simulink model "PCM"  (R2024a)
settings: Solver=VariableStepAuto  StartTime=0.0  StopTime=10.0  RelTol=1e-3
values from neighbouring files (symbols this model uses):
  C = 200*10^(-6)    (= 0.0002)    [Parameters.m]
  ESR = .8    (= 0.8)    [Parameters.m]
  Fs = 10*10^(6)    (= 10000000)    [Parameters.m]
  L = 1*10^(-6)    (= 1e-06)    [Parameters.m]
  Rf = .1    (= 0.1)    [Parameters.m]
  RL = 15*10^(-3)    (= 0.015)    [Parameters.m]
  Rload = 1000    [Parameters.m]
libraries: spsSeriesRLCBranchLib x4, spsMosfetLib x2, spsControlledCurrentSourceLib x1, spsDCVoltageSourceLib x1, simulink_extras x1, spsStairGeneratorLib x1, spsVoltageMeasurementLib x1
settings Model: Creator=User  LastModifiedBy=User

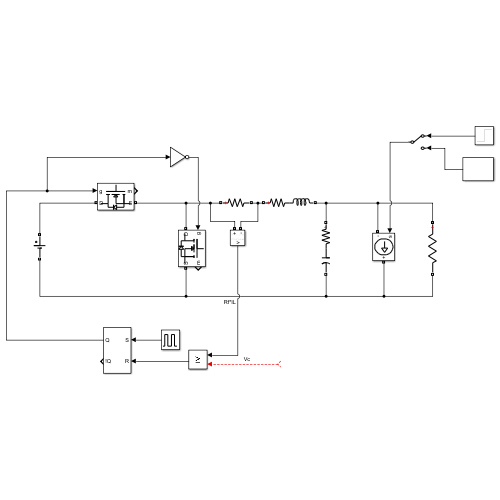
[thumbnail: Simulink's stored preview of the top-level diagram]
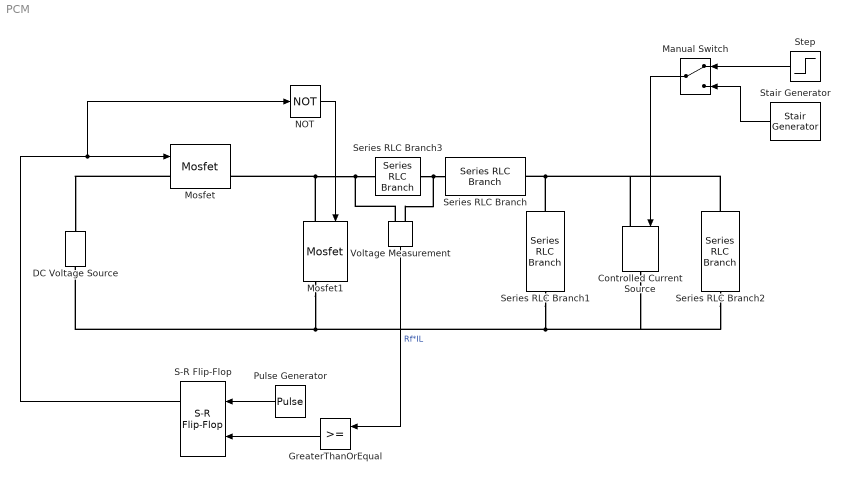
== system PCM ==
  Controlled Current Source : spsControlledCurrentSourceLib/Controlled Current Source  Initialize=on  Source_Type=AC  Amplitude=0  Phase=0  Frequency=0  Measurements=None
  DC Voltage Source : spsDCVoltageSourceLib/DC Voltage Source  Amplitude=5  Measurements=None
  GreaterThanOrEqual : RelationalOperator  OutDataTypeStr=boolean  RndMeth=Simplest  InputSameDT=off
  Manual Switch : ManualSwitch
  Mosfet : spsMosfetLib/Mosfet  Ron=0.1  Lon=0  Rd=0.01  Vfd=0  IC=0  Rs=1e5  Cs=inf  Measurements=on
  Mosfet1 : spsMosfetLib/Mosfet  Ron=0.1  Lon=0  Rd=0.01  Vfd=0  IC=0  Rs=1e5  Cs=inf  Measurements=on
  NOT : Logic  Operator=NOT  IconShape=distinctive  AllPortsSameDT=off  OutDataTypeStr=boolean
  Pulse Generator : DiscretePulseGenerator  PulseType=Time based  Period=1/Fs  PulseWidth=10
  S-R Flip-Flop : simulink_extras/Flip Flops/S-R Flip-Flop  initial_condition=0
  Series RLC Branch : spsSeriesRLCBranchLib/Series RLC Branch  LConnTagsString=__new0  RConnTagsString=__new0  BranchType=RL  Resistance=RL  Inductance=L  SetiL0=off  InitialCurrent=0  Capacitance=1e-6  Setx0=off  InitialVoltage=0  Measurements=None
  Series RLC Branch1 : spsSeriesRLCBranchLib/Series RLC Branch  LConnTagsString=__new0  RConnTagsString=__new0  BranchType=RC  Resistance=ESR  Inductance=L  SetiL0=off  InitialCurrent=0  Capacitance=C  Setx0=off  InitialVoltage=0  Measurements=None
  Series RLC Branch2 : spsSeriesRLCBranchLib/Series RLC Branch  LConnTagsString=__new0  RConnTagsString=__new0  BranchType=R  Resistance=Rload  Inductance=L  SetiL0=off  InitialCurrent=0  Capacitance=1e-6  Setx0=off  InitialVoltage=0  Measurements=None
  Series RLC Branch3 : spsSeriesRLCBranchLib/Series RLC Branch  LConnTagsString=__new0  RConnTagsString=__new0  BranchType=R  Resistance=Rf  Inductance=L  SetiL0=off  InitialCurrent=0  Capacitance=1e-6  Setx0=off  InitialVoltage=0  Measurements=None
  Stair Generator : spsStairGeneratorLib/Stair Generator  t=[0]  e=[5]  Ts=0
  Step : Step  Time=0  Before=5  After=5  SampleTime=0
  Voltage Measurement : spsVoltageMeasurementLib/Voltage Measurement  PhasorSimulation=off  OutputType=Complex  PSBequivalent=0
  wires:
  Stair Generator/1 -> Manual Switch/2
  S-R Flip-Flop/1 -> NOT/1, Mosfet/1
  NOT/1 -> Mosfet1/1
  Pulse Generator/1 -> S-R Flip-Flop/1
  Step/1 -> Manual Switch/1
  Manual Switch/1 -> Controlled Current Source/1
  Voltage Measurement/1 -> GreaterThanOrEqual/1  "Rf*IL"
  GreaterThanOrEqual/1 -> S-R Flip-Flop/2
  ? -> GreaterThanOrEqual/2  "Vc"
  connections:
  Mosfet/LConn1 -- DC Voltage Source/RConn1
  Mosfet1/LConn1 -- Mosfet/RConn1 -- Voltage Measurement/LConn1 -- Series RLC Branch3/LConn1
  Mosfet1/RConn1 -- Controlled Current Source/RConn1 -- Series RLC Branch2/RConn1 -- Series RLC Branch1/RConn1 -- DC Voltage Source/LConn1
  Series RLC Branch1/LConn1 -- Controlled Current Source/LConn1 -- Series RLC Branch2/LConn1 -- Series RLC Branch/RConn1
  Series RLC Branch3/RConn1 -- Voltage Measurement/LConn2 -- Series RLC Branch/LConn1
